simulink model "Bebop8_new_filter_inProgress"  (R2018a)
settings: Solver=VariableStepAuto  StartTime=0.0  StopTime=50  FixedStep=.04  MaxStep=1.00  MinStep=0.005  RelTol=10  AbsTol=10
values from neighbouring files (symbols this model uses):
  flightplan = [dist,0,height,deg2rad(090) ... (first row only)    [compare_cubic_spline_1.m]    (also in initialize_race_realtime.m; initialize_race_realtime_backup_cubic.m; plot_sim.m = [ 4.348, -0.278, height, deg2rad(  0); test_b_spline.m)
  FOV = 1.05    [initialize_race_realtime.m]    (also in initialize_race_realtime_backup_cubic.m)
  g = 9.81    [initialize_race_no_realtime.m]    (also in initialize_race_realtime.m; initialize_race_realtime_backup_cubic.m; moving_average_rls_own.m = P(i-1)*meas*(lambda+meas*P(i-1)*meas)^-1)
  gate_size = 1.4    [initialize_race_realtime.m]    (also in initialize_race_realtime_backup_cubic.m)
  gates = sim_gates(:,:,1)    [eval_sim.m]    (also in initialize_race_realtime.m = [dist,0,height,deg2rad(110); initialize_race_realtime_backup_cubic.m = [dist,0,height,deg2rad(110); plot_sim.m)
  I = [1 0 0 ... (first row only)    [Bebop_sim_init.m]    (also in initialize_race_no_realtime.m; initialize_race_realtime.m; initialize_race_realtime_backup_cubic.m; moving_averge_rls_download.m = ones(1,N))
  init_std_dev = [1.0*ones(1,3),deg2rad(30)]    [initialize_race_realtime.m]    (also in initialize_race_realtime_backup_cubic.m)
  m = 0.68    [calc_plot_spline.m]    (also in calc_spline.m; compare_cubic_spline_1.m = vpasolve(e,r); compare_cubic_spline_2.m = r/3*(-sin(dp)+sqrt(sin(dp)^2-6*cos(dp)+6)); initialize_race_no_realtime.m = 2)
  max_rot_Z = (90)*pi/180    (= 1.57079632679)    [Bebop_sim_init.m]    (also in initialize_race_no_realtime.m = 1.0471975512; initialize_race_realtime.m = 1.0471975512; initialize_race_realtime_backup_cubic.m; run_batch1.m = list_agility(idx_agility)*max_rot_Z)
  max_theta_X = (40)*pi/180    (= 0.698131700798)    [Bebop_sim_init.m]    (also in initialize_race_no_realtime.m = 0.13962634016; initialize_race_realtime.m = 1.308996939; initialize_race_realtime_backup_cubic.m = 1.308996939; run_batch1.m = list_agility(idx_agility)*max_theta_X)
  max_theta_Y = (40)*pi/180    (= 0.698131700798)    [Bebop_sim_init.m]    (also in initialize_race_no_realtime.m = 0.13962634016; initialize_race_realtime.m = 1.308996939; initialize_race_realtime_backup_cubic.m = 1.308996939; run_batch1.m = list_agility(idx_agility)*max_theta_Y)
  max_v_Z = .5    (= 0.5)    [Bebop_sim_init.m]    (also in initialize_race_no_realtime.m = 1; initialize_race_realtime.m = 2; initialize_race_realtime_backup_cubic.m = 3; run_batch1.m = list_agility(idx_agility)*max_v_Z)
  max_vel = 1.0    (= 1)    [initialize_race_realtime.m]    (also in initialize_race_realtime_backup_cubic.m = 1.5; run_batch1.m = list_speed(idx_speed); run_batch2.m = list_speed(idx_speed); run_batch3.m = list_speed(idx_speed))
  spline_init = [P0;P1;P2;P3]    [initialize_race_realtime.m]
  std_dev_factor = 1.0    (= 1)    [initialize_race_realtime.m]
  std_dev_switch = std_dev_factor/5    (= 0.2)    [initialize_race_realtime.m]
undefined symbols (not defined in the file or in its folder): fspecial, gray, Rec, SDTV
libraries: simulink x11, sharedtransform x11, visiontextngfix x7, visionanalysis x7, visiontransforms x3, aerolibactuator x2, aerolibutil x2, visionstatistics x2, visionconversions x2, shared6dof x1, vrlib x1, visionsinks x1
(part 4 of 4)

== matlab function Bebop8_new_filter_inProgress/Guidance/filter_WP_moving_av ==
  data: WP_list_out output; WP_idx_out output; WP_list_in input; WP_idx_in input; WP_std_dev_in input; dist_old_raw input; WP_current_pos input; WP_current_eul input; WP_std_dev_out output; WP_est_out output; WP_P_mat_out output; init_std_dev input; WP_P_mat_in input; WP_est_in input; WP_list_const input
function [WP_list_out, WP_idx_out, WP_std_dev_out, WP_est_out, WP_P_mat_out] = filter_WP(WP_list_in, WP_idx_in, WP_std_dev_in, dist_old_raw, WP_current_pos, WP_current_eul, init_std_dev, WP_P_mat_in, WP_est_in,WP_list_const)
    
%     WP_list_out = zeros(4,4);
%     WP_std_dev_out = zeros(4,1);
    mean_var = [0.3 0.0 0.0 0.0;0.0 0.3 0.0 0.0;0.0 0.0 0.3 0.0;0.0 0.0 0.0 0.3];
    % catch state transition
    WP_idx_out = WP_idx_in;
    if dist_old_raw > 1
        disp('new state')
        WP_idx_out = WP_idx_out+1;
        if WP_idx_out == size(WP_list_in,1)
            WP_idx_out = 0;
        end
        WP_std_dev_in = init_std_dev;
        WP_est_in = WP_list_const(WP_idx_out+1,:)';
        %WP_current_gate_in = WP_list_const(WP_idx_out+1,:)';
        WP_P_mat_in = diag(init_std_dev.^2);
    end
    WP_current_gate = WP_list_const(WP_idx_out+1,:)';
    WP_list_out = WP_list_in;
    
    WP_P_mat_out = WP_P_mat_in;
    WP_std_dev_out = [sqrt(WP_P_mat_out(1,1));
        sqrt(WP_P_mat_out(2,2));
        sqrt(WP_P_mat_out(3,3));
        sqrt(WP_P_mat_out(4,4))];
    
    WP_est_out = WP_est_in;
    
   
    if WP_current_eul(1) > WP_current_gate(4) + pi/2
        euler_used = WP_current_eul(1)-pi;
    elseif WP_current_eul(1) < WP_current_gate(4)-pi/2
        euler_used = WP_current_eul(1)+pi;
    else
        euler_used = WP_current_eul(1);
    end
        
    % check if there is gate information
    if isequal(WP_current_eul, zeros(1,3)) || isequal(WP_current_eul, zeros(3,1))
        % no gate info
        %         disp('gate_global - no corners')
        
    else

        
        if (norm(WP_current_pos(1:2) - WP_current_gate(1:2)) > 2.0) ||...
                WP_current_pos(1) - WP_est_in(1) > 3*sqrt(WP_P_mat_in(1,1)) || ...
                WP_current_pos(2) - WP_est_in(2) > 3*sqrt(WP_P_mat_in(2,2))
                %sqrt(WP_P_mat_in(4,4)) < 0.1 && ...
                %sqrt(WP_P_mat_in(3,3)) < 0.1 && ...
                %sqrt(WP_P_mat_in(2,2)) < 0.1 && ...
                %sqrt(WP_P_mat_in(1,1)) < 0.1) || WP_idx_out ~= WP_idx_out
            %WP_current = [WP_current_pos; WP_current_eul(1)];
            
            %K_gain = WP_P_mat_in*inv(WP_P_mat_in + mean_var);
            
            WP_est_out = WP_est_in;% + K_gain*(WP_current - WP_est_in);
            WP_P_mat_out = WP_P_mat_in;
            
            WP_list_out(WP_idx_out+1,:) = WP_est_out';
            WP_std_dev_out = [sqrt(WP_P_mat_out(1,1));
                sqrt(WP_P_mat_out(2,2));
                sqrt(WP_P_mat_out(3,3));
                sqrt(WP_P_mat_out(4,4))];
            
        else
            
            WP_current = [WP_current_pos; euler_used];
            
            K_gain = WP_P_mat_in*inv(WP_P_mat_in + mean_var);
            
            delta = WP_current-WP_est_in;
            delta(4) = WP_current(4)-WP_est_in(4); %angle_add(WP_current(4),-WP_est_in(4));
            
            WP_est_out(1:3) = WP_est_in(1:3) + K_gain(1:3,:)*(delta);
            WP_est_out(4) = WP_est_in(4) + K_gain(4,:)*delta; %angle_add(WP_est_in(4),K_gain(4,:)*delta);
            WP_P_mat_out = (eye(4) - K_gain)*WP_P_mat_in;
            
            WP_list_out(WP_idx_out+1,:) = WP_est_out';
            WP_std_dev_out = [sqrt(WP_P_mat_out(1,1));
                sqrt(WP_P_mat_out(2,2));
                sqrt(WP_P_mat_out(3,3));
                sqrt(WP_P_mat_out(4,4))];
        end

%         lambda = 0.1;
%         
%         WP_average = WP_list_out(WP_idx_out+1,:)';
%         
%        
%         delta = WP_current-WP_average;
%         delta(4) = angle_add(WP_current(4),-WP_average(4));
%         std = abs(delta) ./ sqrt(WP_std_dev_out);
%     
%         alpha = lambda.^(2*std);
%         alpha = min(alpha, lambda);
% %         alpha = max(alpha, 0.001);
%         WP_average(1:3) = WP_average(1:3) + alpha(1:3).*delta(1:3);
%         WP_average(4) = angle_add(WP_average(4),alpha(4)*delta(4));
%         
%         WP_std_dev_out = sqrt((1-alpha).*(WP_std_dev_out.^2+alpha.*delta.*delta));
% 
%         WP_list_out(WP_idx_out+1,:) = WP_average;
        
    end
end

function sum = angle_add(a1,a2)
    sum = atan2(sin(a1+a2),cos(a1+a2));
end



% 
%         if norm(WP_current_pos' - WP_average_pos) < 0.7
%             WP_average_pos = alpha*WP_current_pos' + (1-alpha)*WP_average_pos;
%             WP_current_hdg = WP_current_ori(1);
%             WP_average_hdg = atan2(alpha*sin(WP_current_hdg) + (1-alpha)*sin(WP_average_hdg), ...
%                 alpha*cos(WP_current_hdg) + (1-alpha)*cos(WP_average_hdg));
%             WP_average = [WP_average_pos, WP_average_hdg];
%             WP_list_out(state0_out+1,:) = WP_average;
%         end

== matlab function Bebop8_new_filter_inProgress/Vision System/gate_global ==
  data: tVec input; rMat input; drone_pos input; drone_ori input; gate_pos_global output; gate_eul_global output
function [gate_pos_global, gate_eul_global]  = gate_global(tVec, rMat, drone_pos, drone_ori)

    gate_pos_global = zeros(3,1);
    gate_eul_global = zeros(3,1);
%     drone_rotm = axang2rotm(drone_ori');
%     gate_pos_local = quatrotate(drone_q,gate_pos_cam);
%     gate_pos_local = drone_rotm * gate_pos_cam';
%     gate_pos_global = gate_pos_local + drone_pos';
%     gate_pos_global = gate_pos_local;

if isequal(tVec,zeros(1,3))
%     disp('gate_global - no corners')
    return
end
    
    %% drone pos
    drone_pos;
    
    %% drone orientation
    dRg = eul2rotm([drone_ori(3),drone_ori(2),drone_ori(1)]);
    
    %% convert gate pos
    % tVec = right down front, drone was front left up
    dRc = eul2rotm([pi/2,-pi/2,0],'ZYX');
    cRd = dRc^-1;
    cRg = dRg*cRd;
    rel= cRg*tVec';
    gate_pos_global = drone_pos + rel;
    
    % rel = -dRs*tvec';
    % gate_pos_global = drone_pos + rel';
    
    %% convert gate orientation
    rot = squeeze(rMat);
    extra = eul2rotm([0,pi/2,0],'ZYX');
    gate_rot = dRg*cRd*rot^-1*extra;
    gate_eul_global = rotm2eul(gate_rot)';
%     
%     wRc = rMat;
%     one_more = 1;%eul2rotm([pi,0,-pi/2]);
%     another_one = 1;%eul2rotm([pi/2,0,0]);
%     wRs = another_one*one_more*cRg*wRc;
%     
%     gate_ori_global = (rotm2eul(wRs))';

%       rot = rMat*cRg^-1;
%       gate_yaw=rotm2eul(rot);
    
end
